simulink model "landingSimulation"  (R2016a)
settings: Solver=FixedStepAuto  StartTime=0.0  StopTime=60.0  FixedStep=0.001  RelTol=1e-3
settings Model: Creator=jason  LastModifiedBy=jason

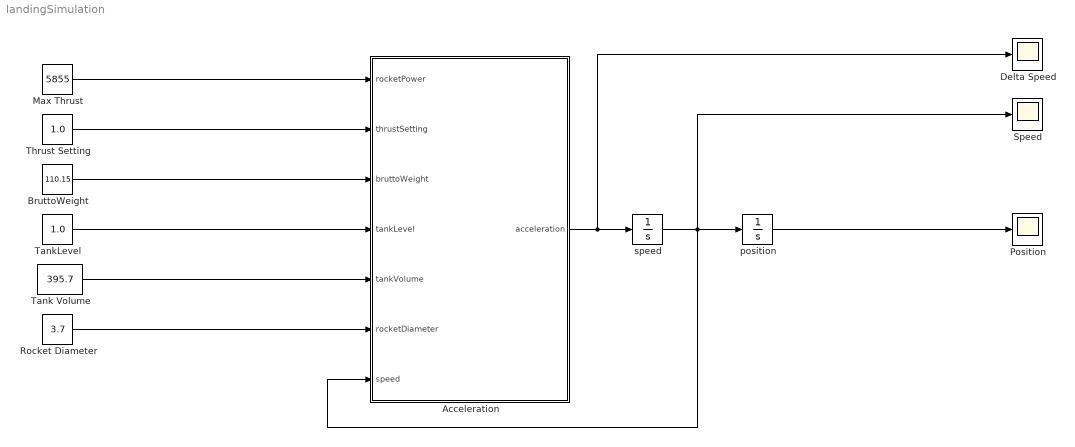
== system landingSimulation ==
  Acceleration : MATLAB Function  TreatAsAtomicUnit=on
  BruttoWeight : Constant  Value=110.15
  Delta Speed : Scope
  Max Thrust : Constant  Value=5855
  Position : Scope
  Rocket Diameter : Constant  Value=3.7
  Speed : Scope
  Tank Volume : Constant  Value=395.7
  TankLevel : Constant  Value=1.0
  Thrust Setting : Constant  Value=1.0
  position : Integrator
  speed : Integrator
  wires:
  speed/1 -> Speed/1, position/1, Acceleration/7(speed)
  Rocket Diameter/1 -> Acceleration/6(rocketDiameter)
  position/1 -> Position/1
  Thrust Setting/1 -> Acceleration/2(thrustSetting)
  Acceleration/1(acceleration) -> Delta Speed/1, speed/1
  Max Thrust/1 -> Acceleration/1(rocketPower)
  BruttoWeight/1 -> Acceleration/3(bruttoWeight)
  TankLevel/1 -> Acceleration/4(tankLevel)
  Tank Volume/1 -> Acceleration/5(tankVolume)

== matlab function landingSimulation/Acceleration ==
  data: rocketPower input; thrustSetting input; bruttoWeight input; tankLevel input; tankVolume input; rocketDiameter input; acceleration output; speed input
function acceleration = Acceleration( rocketPower, thrustSetting, bruttoWeight, tankLevel, tankVolume, rocketDiameter, speed )
    mass = Mass(bruttoWeight, tankLevel, tankVolume);

    thrust = Thrust(thrustSetting, rocketPower, mass);
    gravity = Gravity();
    airDrag = AirDrag(speed, rocketDiameter, mass);
    
    acceleration = thrust - gravity + airDrag;
end
